simulink model "test"  (Simulink 7.9)
settings: Solver=ode45  StartTime=0.0  StopTime=10.0  RelTol=1e-8
values from neighbouring files (symbols this model uses):
  zeta_command = [0,0.,0,0,0.3,0,0.3,0,0.6,0,0.4,0]    [kinematic_parameters.m]
undefined symbols (not defined in the file or in its folder): initial_ee_pose
settings Model: Creator=simena  LastModifiedBy=simena

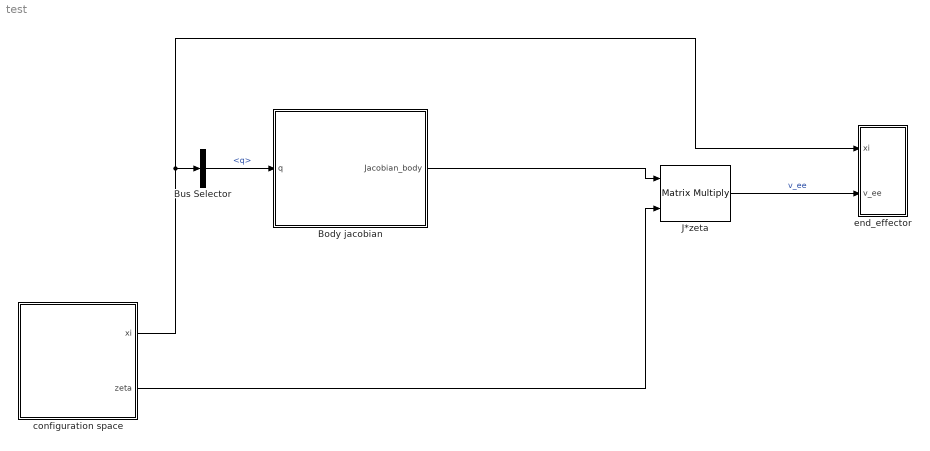
== system test ==
  Body jacobian : MATLAB Function  TreatAsAtomicUnit=on
  Bus Selector : BusSelector  OutputSignals=q
  J*zeta : Product  Multiplication=Matrix(*)  RndMeth=Zero
  configuration space : Subsystem
  end_effector : Subsystem
  wires:
  Body jacobian/1(Jacobian_body) -> J*zeta/1
  configuration space/1(xi) -> Bus Selector/1, end_effector/1(xi)
  Bus Selector/1 -> Body jacobian/1(q)  "<q>"
  J*zeta/1 -> end_effector/2(v_ee)  "v_ee"
  configuration space/2(zeta) -> J*zeta/2

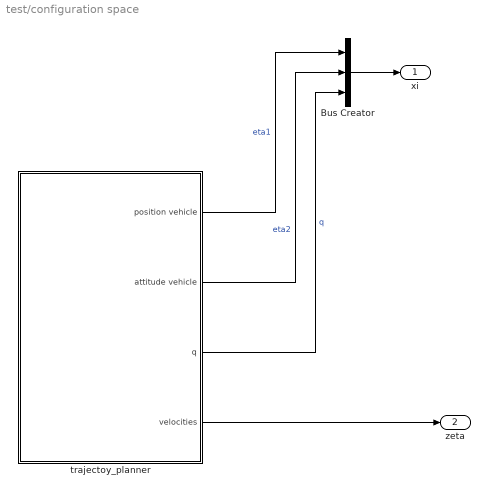
== system test/configuration space ==
  Bus Creator : BusCreator  Inputs=3
  trajectoy_planner : Subsystem
  xi : Outport
  zeta : Outport  Port=2
  wires:
  trajectoy_planner/1(position vehicle) -> Bus Creator/1  "eta1"
  trajectoy_planner/2(attitude vehicle) -> Bus Creator/2  "eta2"
  trajectoy_planner/3(q) -> Bus Creator/3  "q"
  trajectoy_planner/4(velocities) -> zeta/1
  Bus Creator/1 -> xi/1

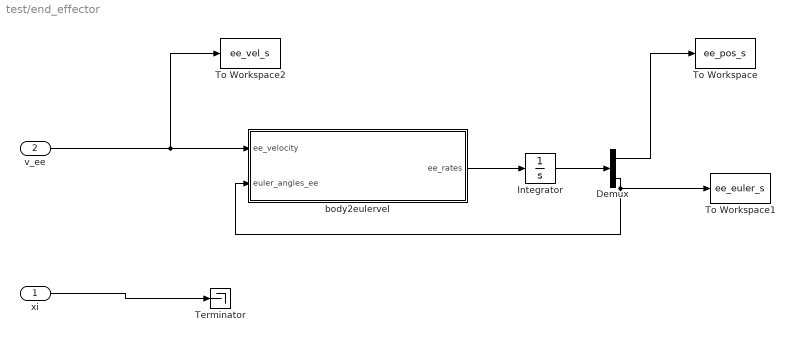
== system test/end_effector ==
  xi : Inport
  v_ee : Inport  Port=2
  Demux : Demux  Outputs=2
  Integrator : Integrator  InitialCondition=initial_ee_pose
  Terminator : Terminator
  To Workspace : ToWorkspace  VariableName=ee_pos_s  SampleTime=-1  SaveFormat=Structure With Time
  To Workspace1 : ToWorkspace  VariableName=ee_euler_s  SampleTime=-1  SaveFormat=Structure With Time
  To Workspace2 : ToWorkspace  VariableName=ee_vel_s  SampleTime=-1  SaveFormat=Structure With Time
  body2eulervel : MATLAB Function  TreatAsAtomicUnit=on
  wires:
  v_ee/1 -> body2eulervel/1(ee_velocity), To Workspace2/1
  body2eulervel/1(ee_rates) -> Integrator/1
  Integrator/1 -> Demux/1
  Demux/1 -> To Workspace/1
  Demux/2 -> body2eulervel/2(euler_angles_ee), To Workspace1/1
  xi/1 -> Terminator/1

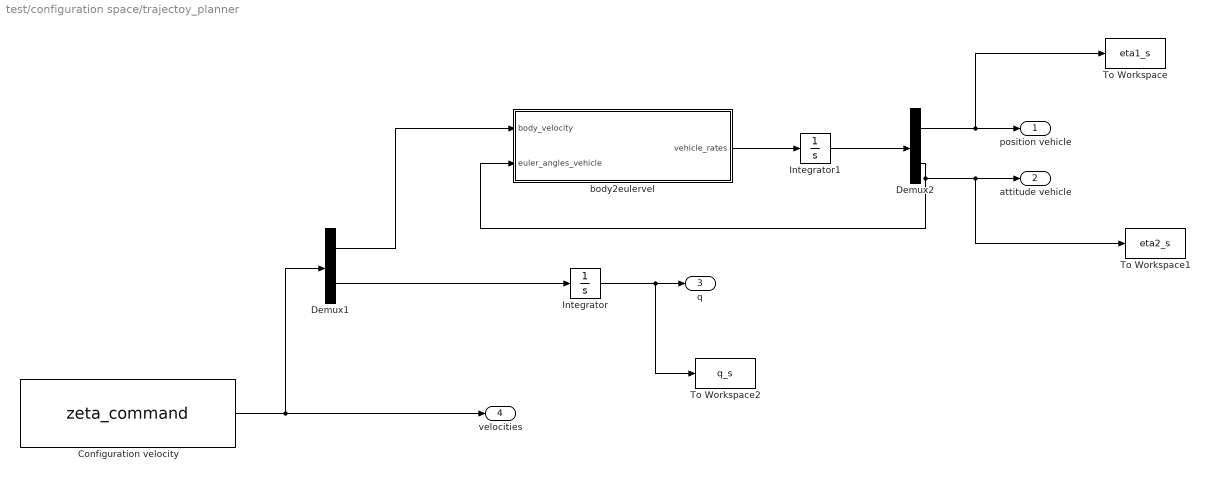
== system test/configuration space/trajectoy_planner ==
  "Configuration velocity " : Constant  Value=zeta_command
  Demux1 : Demux  Outputs=2
  Demux2 : Demux  Outputs=2
  Integrator : Integrator
  Integrator1 : Integrator
  To Workspace : ToWorkspace  VariableName=eta1_s  SampleTime=-1  SaveFormat=Structure With Time
  To Workspace1 : ToWorkspace  VariableName=eta2_s  SampleTime=-1  SaveFormat=Structure With Time
  To Workspace2 : ToWorkspace  VariableName=q_s  SampleTime=-1  SaveFormat=Structure With Time
  body2eulervel : MATLAB Function  TreatAsAtomicUnit=on
  position vehicle : Outport
  attitude vehicle : Outport  Port=2
  q : Outport  Port=3
  velocities : Outport  Port=4
  wires:
  "Configuration velocity "/1 -> velocities/1, Demux1/1
  Demux1/2 -> Integrator/1
  Demux1/1 -> body2eulervel/1(body_velocity)
  Integrator/1 -> q/1, To Workspace2/1
  body2eulervel/1(vehicle_rates) -> Integrator1/1
  Integrator1/1 -> Demux2/1
  Demux2/2 -> body2eulervel/2(euler_angles_vehicle), attitude vehicle/1, To Workspace1/1
  Demux2/1 -> position vehicle/1, To Workspace/1

== matlab function end_effector/body2eulervel ==
  data: ee_velocity input double; ee_rates output double; euler_angles_ee input double
function ee_rates = fcn(ee_velocity, euler_angles_ee)                       
    %#codegen
    coder.extrinsic('analytical_jacobian');
    J=analytical_jacobian(euler_angles_ee);

    ee_rates = zeros(6,1);
    ee_rates=J*ee_velocity;
end

== matlab function Body jacobian ==
  data: q input double; Jacobian_body output double
function Jacobian_body = fcn(q)
    %#codegen
    Jacobian_body=zeros(6,12);
    coder.extrinsic('body_jacobian');
    newq=zeros(1,6);
    newq=q;
    Jacobian_body=body_jacobian(newq);
end

== matlab function configuration space/trajectoy_planner/body2eulervel ==
  data: body_velocity input double; vehicle_rates output double; euler_angles_vehicle input double
function vehicle_rates = fcn(body_velocity, euler_angles_vehicle)                       
    %#codegen
    coder.extrinsic('analytical_jacobian');
    J=analytical_jacobian(euler_angles_vehicle);

    vehicle_rates = zeros(6,1);
    vehicle_rates=J*body_velocity;
end
